simulink model "problem12"  (R2021a)
settings: Solver=VariableStepAuto  StartTime=0.0  StopTime=10.0  RelTol=1e-3
undefined symbols (not defined in the file): B, J1, J2, J3, J4, Kd_1, Kd_2, Kd_3, Kd_4, Kp_1, Kp_2, Kp_3, Kp_4, qr_1, qr_2, qr_3, qr_4, T_L
settings Model: Creator=Luky  LastModifiedBy=Luky
settings SolverCC: AlgebraicLoopSolver=TrustRegion
settings DataIOCC: Refine=50

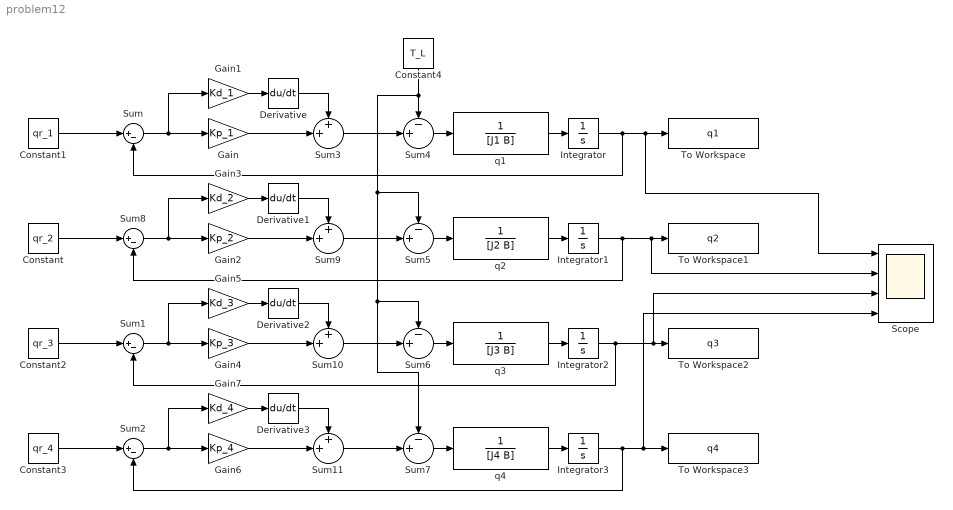
== system problem12 ==
  Constant : Constant  Value=qr_2
  Constant1 : Constant  Value=qr_1
  Constant2 : Constant  Value=qr_3
  Constant3 : Constant  Value=qr_4
  Constant4 : Constant  Value=T_L
  Derivative{,1..3} (4 alike) : Derivative
  Gain : Gain  Gain=Kp_1
  Gain1 : Gain  Gain=Kd_1
  Gain2 : Gain  Gain=Kp_2
  Gain3 : Gain  Gain=Kd_2
  Gain4 : Gain  Gain=Kp_3
  Gain5 : Gain  Gain=Kd_3
  Gain6 : Gain  Gain=Kp_4
  Gain7 : Gain  Gain=Kd_4
  Integrator{,1..3} (4 alike) : Integrator
  Scope : Scope  NumInputPorts=4
  Sum{,1..2,8} (4 alike) : Sum  Inputs=|+-
  Sum{3,9..11} (4 alike) : Sum  Inputs=++|
  Sum{4..7} (4 alike) : Sum  Inputs=-+|
  To Workspace : ToWorkspace  VariableName=q1  SaveFormat=Timeseries  SampleTime=-1
  To Workspace1 : ToWorkspace  VariableName=q2  SaveFormat=Timeseries  SampleTime=-1
  To Workspace2 : ToWorkspace  VariableName=q3  SaveFormat=Timeseries  SampleTime=-1
  To Workspace3 : ToWorkspace  VariableName=q4  SaveFormat=Timeseries  SampleTime=-1
  q1 : TransferFcn  Denominator=[J1 B]
  q2 : TransferFcn  Denominator=[J2 B]
  q3 : TransferFcn  Denominator=[J3 B]
  q4 : TransferFcn  Denominator=[J4 B]
  wires:
  q1/1 -> Integrator/1
  q2/1 -> Integrator1/1
  q3/1 -> Integrator2/1
  q4/1 -> Integrator3/1
  Sum/1 -> Gain1/1, Gain/1
  Constant1/1 -> Sum/1
  Constant/1 -> Sum8/1
  Constant2/1 -> Sum1/1
  Sum3/1 -> Sum4/2
  Sum4/1 -> q1/1
  Sum6/1 -> q3/1
  Sum5/1 -> q2/1
  Sum7/1 -> q4/1
  Integrator/1 -> Sum/2, Scope/1, To Workspace/1
  Integrator1/1 -> Sum8/2, Scope/2, To Workspace1/1
  Integrator2/1 -> Sum1/2, Scope/3, To Workspace2/1
  Integrator3/1 -> Sum2/2, Scope/4, To Workspace3/1
  Gain1/1 -> Derivative/1
  Derivative/1 -> Sum3/1
  Gain/1 -> Sum3/2
  Derivative1/1 -> Sum9/1
  Gain3/1 -> Derivative1/1
  Gain2/1 -> Sum9/2
  Sum8/1 -> Gain3/1, Gain2/1
  Sum9/1 -> Sum5/2
  Derivative2/1 -> Sum10/1
  Gain5/1 -> Derivative2/1
  Gain4/1 -> Sum10/2
  Sum1/1 -> Gain5/1, Gain4/1
  Sum10/1 -> Sum6/2
  Derivative3/1 -> Sum11/1
  Gain7/1 -> Derivative3/1
  Gain6/1 -> Sum11/2
  Sum2/1 -> Gain7/1, Gain6/1
  Sum11/1 -> Sum7/2
  Constant3/1 -> Sum2/1
  Constant4/1 -> Sum5/1, Sum6/1, Sum7/1, Sum4/1
